simulink model "cruise_ctrl_kpit"  (Simulink 7.5)
settings: Solver=ode45  StartTime=0.0  StopTime=60  MaxStep=0.1  RelTol=1e-3
PreLoadFcn:
  | m = 1000;
  | gear_ratio= [40, 25, 16, 12, 10];
  | Tm = 190;
  | wm = 420;
  | beta = 0.4;
  | croll= 0.01;
  | air_density= 1.3;
  | Cd = 0.32;
  | A = 2.4;
  | g = 9.8;
  | theta = 0;
  | gear = 3;
settings Model: Creator=Cole Lepine  LastModifiedBy=User
settings OptimizationCC: InitFltsAndDblsToZero=on
settings DebuggingCC: StrictBusMsg=Warning
settings RTWCC: GenerateReport=on  LaunchReport=on

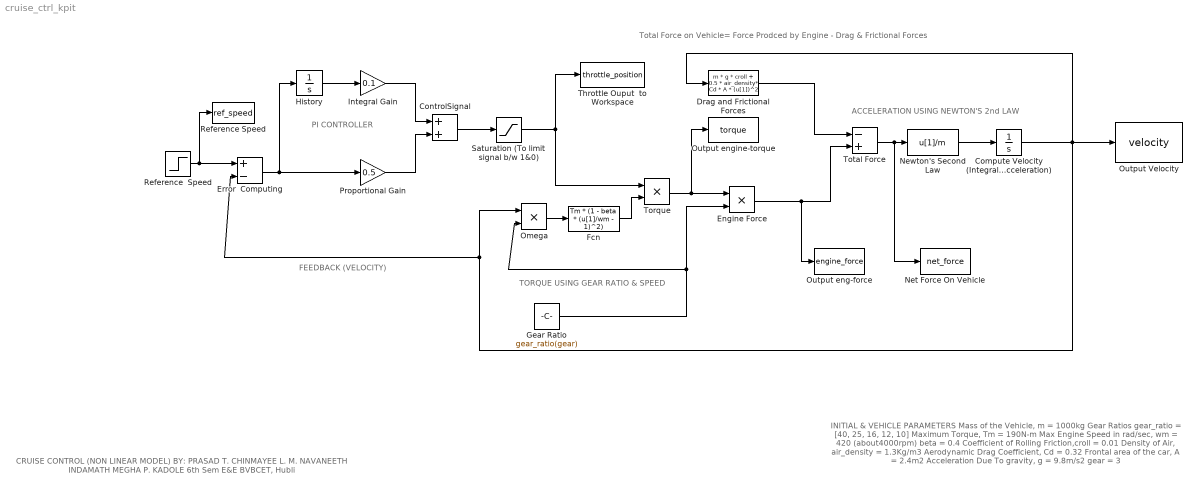
== system cruise_ctrl_kpit ==
  note: PI CONTROLLER
  note: TORQUE USING GEAR RATIO & SPEED
  note: ACCELERATION USING
      |  NEWTON'S 2nd LAW
  note: Total Force on Vehicle=
      | Force Prodced by Engine - Drag & Frictional Forces
  note: FEEDBACK (VELOCITY)
  note: INITIAL & VEHICLE PARAMETERS
      | Mass of the Vehicle, m = 1000kg
      | Gear Ratios gear_ratio = [40, 25, 16, 12, 10]
      | Maximum Torque, Tm = 190N-m
      | Max Engine Speed in rad/sec, wm = 420 (about4000rpm)
      | beta = 0.4
      | Coefficient of Rolling Friction,croll = 0.01
      | Density of Air, air_density = 1.3Kg/m3
      | Aerodynamic Drag Coefficient, Cd = 0.32
      |  Frontal area of the car, A = 2.4m2
      | Acceleration Due To gravity, g = 9.8m/s2
      | gear = 3
  note: CRUISE CONTROL (NON LINEAR MODEL)
      | BY: PRASAD T.
      | CHINMAYEE L. M.
      | NAVANEETH  INDAMATH
      | MEGHA P. KADOLE
      | 6th Sem E&E BVBCET, Hubli
  Compute Velocity (Integral of Acceleration) : Integrator  InitialCondition=20
  ControlSignal : Sum  OutDataType=sfix(16)  OutScaling=2^-10
  Drag and Frictional Forces : Fcn  Expr=m * g * croll + 0.5 * air_density* Cd * A * (u[1])^2
  Engine Force : Product  Inputs=**  OutDataType=sfix(16)  OutScaling=2^-10
  Error  Computing : Sum  Inputs=+-  OutDataType=sfix(16)  OutScaling=2^-10
  Fcn : Fcn  Expr=Tm * (1 - beta * (u[1]/wm - 1)^2)
  Gear Ratio : Constant  Value=gear_ratio(gear)  OutDataType=sfix(16)  OutScaling=2^0
  History : Integrator  InitialCondition=1
  Integral Gain : Gain  Gain=0.1  ParameterDataType=sfix(16)  ParameterScaling=2^0  OutDataType=sfix(16)  OutScaling=2^0
  Net Force On Vehicle : ToWorkspace  VariableName=net_force  SampleTime=-1  SaveFormat=Array
  Newton's Second Law : Fcn  Expr=u[1]/m
  Omega : Product  OutDataType=sfix(16)  OutScaling=2^0  RndMeth=Zero
  Output Velocity : ToWorkspace  VariableName=velocity  SampleTime=-1  SaveFormat=Array
  Output eng-force : ToWorkspace  VariableName=engine_force  SampleTime=-1  SaveFormat=Array
  Output engine-torque : ToWorkspace  VariableName=torque  SampleTime=-1  SaveFormat=Array
  Proportional Gain : Gain  Gain=0.5  ParameterDataType=sfix(16)  ParameterScaling=2^0  OutDataType=sfix(16)  OutScaling=2^0
  Reference  Speed : Step  Time=20  Before=20  After=30  SampleTime=0
  Reference Speed : ToWorkspace  VariableName=ref_speed  SampleTime=-1  SaveFormat=Array
  Saturation (To limit signal b/w 1&0) : Saturate  UpperLimit=1  LowerLimit=0  OutDataType=sfix(16)  OutScaling=2^0
  Throttle Ouput  to Workspace : ToWorkspace  VariableName=throttle_position  SampleTime=-1  SaveFormat=Array
  Torque : Product  OutDataType=sfix(16)  OutScaling=2^0  RndMeth=Zero
  Total Force : Sum  Inputs=-+  OutDataType=sfix(16)  OutScaling=2^-10
  wires:
  Engine Force/1 -> Total Force/2, Output eng-force/1
  Total Force/1 -> Net Force On Vehicle/1, Newton's Second Law/1
  Newton's Second Law/1 -> Compute Velocity (Integral of Acceleration)/1
  Compute Velocity (Integral of Acceleration)/1 -> Omega/1, Error  Computing/2, Output Velocity/1, Drag and Frictional Forces/1
  Gear Ratio/1 -> Engine Force/2, Omega/2
  Omega/1 -> Fcn/1
  Torque/1 -> Engine Force/1, Output engine-torque/1
  Fcn/1 -> Torque/2
  Saturation (To limit signal b/w 1&0)/1 -> Throttle Ouput  to Workspace/1, Torque/1
  Reference  Speed/1 -> Error  Computing/1, Reference Speed/1
  ControlSignal/1 -> Saturation (To limit signal b/w 1&0)/1
  Proportional Gain/1 -> ControlSignal/2
  Integral Gain/1 -> ControlSignal/1
  Error  Computing/1 -> Proportional Gain/1, History/1
  History/1 -> Integral Gain/1
  Drag and Frictional Forces/1 -> Total Force/1
